simulink model "CLIK_trasp_jacob_1order"  (R2021a)
settings: Solver=VariableStepAuto  StartTime=0.0  StopTime=50  RelTol=1e-3
values from neighbouring files (symbols this model uses):
  K = diag([1000 10 100])    [pseudo_traiettoria.m]
  q0 = scara.ikine(T0, 'mask', [1 1 1 1 0 0])    [pseudo_traiettoria.m]    (also in traiettoria.m)
  Tc = 0.001    [pseudo_traiettoria.m]    (also in traiettoria.m)
undefined symbols (not defined in the file or in its folder): DiscIntNeverNeededParam
settings Model: Creator=ciro  LastModifiedBy=Ciro

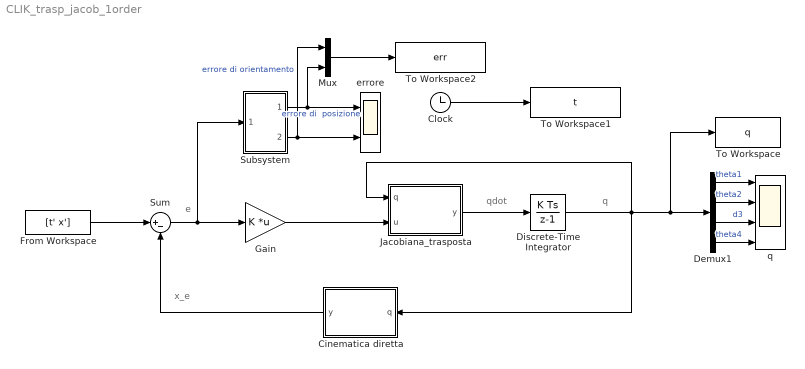
== system CLIK_trasp_jacob_1order ==
  note: qdot
  note: q
  note: e
  note: x_e
  Cinematica diretta : MATLAB Function  TreatAsAtomicUnit=on
  Clock : Clock
  Demux1 : Demux
  Discrete-Time Integrator : DiscreteIntegrator  InitialCondition=q0  SampleTime=Tc  ICPrevOutput=DiscIntNeverNeededParam  ICPrevScaledInput=DiscIntNeverNeededParam
  From Workspace : FromWorkspace  VariableName=[t' x']  OutDataTypeStr=double  SampleTime=Tc  OutputAfterFinalValue=Holding final value
  Gain : Gain  Gain=K  Multiplication=Matrix(K*u)
  Jacobiana_trasposta : MATLAB Function  TreatAsAtomicUnit=on
  Mux : Mux  Inputs=2
  Subsystem : Subsystem
  Sum : Sum  Inputs=|+-
  To Workspace : ToWorkspace  VariableName=q  SampleTime=Tc
      settings: Save2DSignal=2-D array (concatenate along first dimension)
  To Workspace1 : ToWorkspace  VariableName=t  SampleTime=Tc
      settings: Save2DSignal=2-D array (concatenate along first dimension)
  To Workspace2 : ToWorkspace  VariableName=err  SampleTime=-1
      settings: Save2DSignal=2-D array (concatenate along first dimension)
  errore : Scope  NumInputPorts=2
  q : Scope  NumInputPorts=4
  wires:
  From Workspace/1 -> Sum/1
  Sum/1 -> Subsystem/1(In1), Gain/1
  Gain/1 -> Jacobiana_trasposta/2(u)
  Jacobiana_trasposta/1(y) -> Discrete-Time Integrator/1
  Discrete-Time Integrator/1 -> To Workspace/1, Demux1/1, Cinematica diretta/1(q), Jacobiana_trasposta/1(q)
  Cinematica diretta/1(y) -> Sum/2
  Demux1/1 -> q/1  "theta1"
  Demux1/2 -> q/2  "theta2"
  Demux1/3 -> q/3  "d3"
  Demux1/4 -> q/4  "theta4"
  Clock/1 -> To Workspace1/1
  Subsystem/1(Out1) -> Mux/2, errore/1  "errore di  posizione"
  Subsystem/2(Out2) -> Mux/1, errore/2  "errore di orientamento"
  Mux/1 -> To Workspace2/1

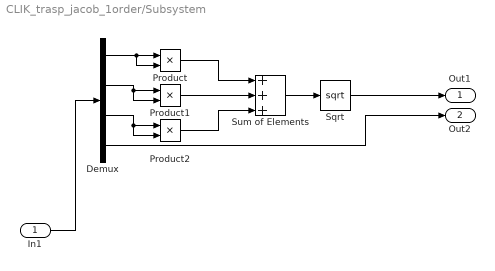
== system CLIK_trasp_jacob_1order/Subsystem ==
  In1 : Inport
  Demux : Demux
  Product : Product
  Product1 : Product
  Product2 : Product
  Sqrt : Sqrt  SaturateOnIntegerOverflow=on
  Sum of Elements : Sum  Inputs=+++
  Out1 : Outport
  Out2 : Outport  Port=2
  wires:
  Product/1 -> Sum of Elements/1
  Sum of Elements/1 -> Sqrt/1
  Demux/2 -> Product1/2, Product1/1
  Demux/1 -> Product/2, Product/1
  Demux/3 -> Product2/2, Product2/1
  Product1/1 -> Sum of Elements/2
  Demux/4 -> Out2/1
  Sqrt/1 -> Out1/1
  Product2/1 -> Sum of Elements/3
  In1/1 -> Demux/1

== matlab function CLIK_trasp_jacob_1order/Jacobiana_trasposta ==
  data: q input; u input; y output
function y = fcn(q, u)

J = [ -0.5*(sin(q(1))+sin(q(1)+q(2))) -0.5*sin(q(1)+q(2)) 0 0;
       0.5*(cos(q(1))+cos(q(1)+q(2)))  0.5*cos(q(1)+q(2)) 0 0;
       0                               0                 -1 0;
       1                               1                  0 -1];
   
y = (J')*u;

== matlab function CLIK_trasp_jacob_1order/Cinematica diretta ==
  data: q input; y output
function y = fcn(q)

xe = [0.5*(cos(q(1))+cos(q(1)+q(2)));
      0.5*(sin(q(1))+sin(q(1)+q(2)));
      0.8-q(3);
      q(1)+q(2)-q(4)];

y = xe;
